simulink model "CIMA_LQ"  (R2023b)
settings: Solver=VariableStepAuto  StartTime=0.0  StopTime=30  RelTol=1e-6
values from neighbouring files (symbols this model uses):
  A = J_eq    [CIMA_Control_routine.m]
  a = 10    [CIMA_Classification_Stab_Equilibrium.m]    (also in CIMA_Control_routine.m)
  B = [1;0]    [CIMA_Control_routine.m]
  b = b_vec(i)    [CIMA_Classification_Stab_Equilibrium.m]    (also in CIMA_Control_routine.m = 2)
  C = eye(2)    [CIMA_Control_routine.m]
  D = zeros(2,1)    [CIMA_Control_routine.m]
  Eq = [x1_eq;x2_eq]    [CIMA_Control_routine.m]
  Ki = K(3)    [CIMA_Control_routine.m]
  Kp = K(1:2)    [CIMA_Control_routine.m]
  x0 = [x1_eq+0.5; x2_eq+0.2]    [CIMA_Control_routine.m]
settings Model: Creator=user  LastModifiedBy=user

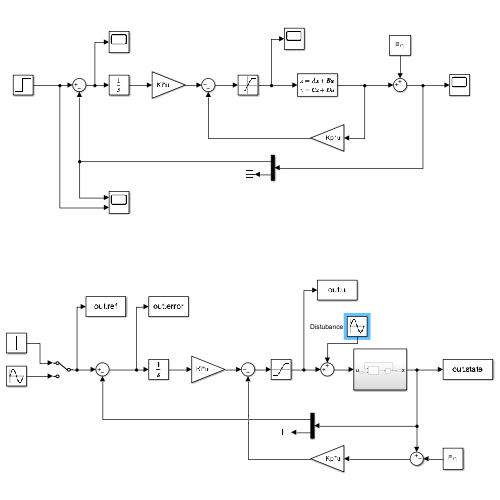
[thumbnail: Simulink's stored preview of the top-level diagram]
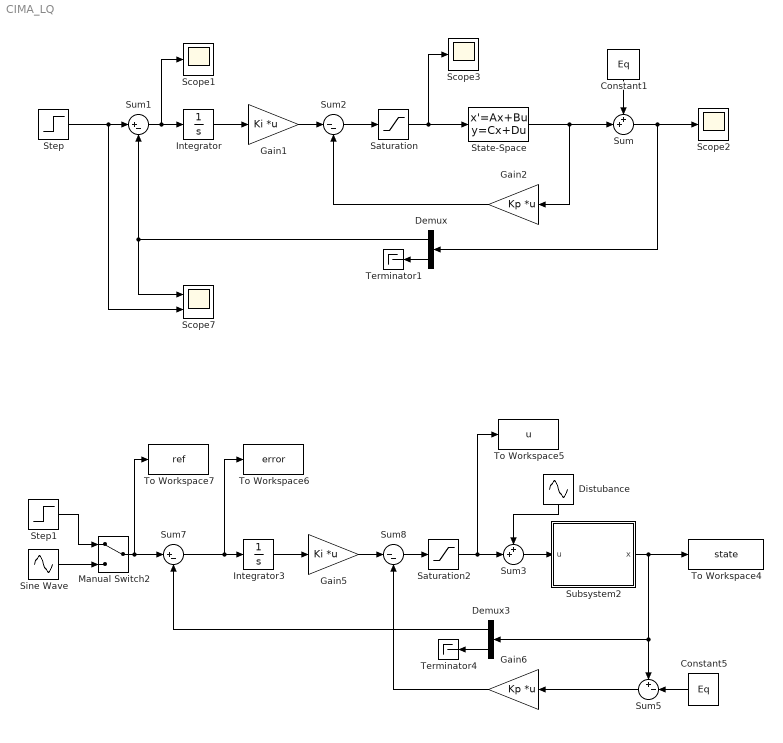
== system CIMA_LQ ==
  Constant1 : Constant  Value=Eq
  Constant5 : Constant  Value=Eq
  Demux : Demux  Outputs=2
  Demux3 : Demux  Outputs=2
  Distubance : Sin  Amplitude=0.3*0  SampleTime=0
  Gain1 : Gain  Gain=Ki  Multiplication=Matrix(K*u)
  Gain2 : Gain  Gain=Kp  Multiplication=Matrix(K*u)
  Gain5 : Gain  Gain=Ki  Multiplication=Matrix(K*u)
  Gain6 : Gain  Gain=Kp  Multiplication=Matrix(K*u)
  Integrator : Integrator
  Integrator3 : Integrator
  Manual Switch2 : ManualSwitch
  Saturation : Saturate  UpperLimit=20  LowerLimit=0
  Saturation2 : Saturate  UpperLimit=20  LowerLimit=0
  Scope1 : Scope
  Scope2 : Scope
  Scope3 : Scope
  Scope7 : Scope  NumInputPorts=2
  Sine Wave : Sin  Amplitude=0.5  Bias=5  Frequency=2  SampleTime=0
  State-Space : StateSpace  A=A  B=B  C=C  D=D  InitialCondition=x0-Eq  ParameterTunability=Optimized
  Step : Step  Time=0  After=5  SampleTime=0
  Step1 : Step  Time=0  After=5  SampleTime=0
  Subsystem2 : Subsystem
  Sum : Sum  Inputs=++|
  Sum1 : Sum  Inputs=|+-
  Sum2 : Sum  Inputs=|--
  Sum3 : Sum  Inputs=++|
  Sum5 : Sum  Inputs=+-|
  Sum7 : Sum  Inputs=|+-
  Sum8 : Sum  Inputs=|--
  Terminator1 : Terminator
  Terminator4 : Terminator
  To Workspace4 : ToWorkspace  VariableName=state  SaveFormat=Structure With Time  SampleTime=-1
  To Workspace5 : ToWorkspace  VariableName=u  SaveFormat=Structure With Time  SampleTime=-1
  To Workspace6 : ToWorkspace  VariableName=error  SaveFormat=Structure With Time  SampleTime=-1
  To Workspace7 : ToWorkspace  VariableName=ref  SaveFormat=Structure With Time  SampleTime=-1
  wires:
  Integrator/1 -> Gain1/1
  Sum2/1 -> Saturation/1
  Demux/1 -> Sum1/2, Scope7/1
  Gain1/1 -> Sum2/1
  Gain2/1 -> Sum2/2
  Sum/1 -> Scope2/1, Demux/1
  Sum1/1 -> Scope1/1, Integrator/1
  Demux/2 -> Terminator1/1
  Step/1 -> Scope7/2, Sum1/1
  Constant1/1 -> Sum/1
  State-Space/1 -> Gain2/1, Sum/2
  Saturation/1 -> State-Space/1, Scope3/1
  Demux3/1 -> Sum7/2
  Gain5/1 -> Sum8/1
  Gain6/1 -> Sum8/2
  Sum8/1 -> Saturation2/1
  Demux3/2 -> Terminator4/1
  Sum7/1 -> To Workspace6/1, Integrator3/1
  Manual Switch2/1 -> To Workspace7/1, Sum7/1
  Integrator3/1 -> Gain5/1
  Saturation2/1 -> To Workspace5/1, Sum3/2
  Step1/1 -> Manual Switch2/1
  Sine Wave/1 -> Manual Switch2/2
  Sum5/1 -> Gain6/1
  Constant5/1 -> Sum5/2
  Sum3/1 -> Subsystem2/1(u)
  Distubance/1 -> Sum3/1
  Subsystem2/1(x) -> To Workspace4/1, Demux3/1, Sum5/1

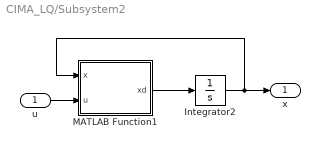
== system CIMA_LQ/Subsystem2 ==
  u : Inport
  Integrator2 : Integrator  InitialCondition=x0  UpperSaturationLimit=18
  MATLAB Function1 : MATLAB Function  TreatAsAtomicUnit=on
  x : Outport
  wires:
  MATLAB Function1/1(xd) -> Integrator2/1
  Integrator2/1 -> x/1, MATLAB Function1/1(x)
  u/1 -> MATLAB Function1/2(u)

== matlab function CIMA_LQ/Subsystem2/MATLAB Function1 ==
  data: x input; u input; xd output; a parameter; b parameter
function xd = cima(x, u, a, b)

xd1 = a -x(1) - 4*x(1)*x(2)/(1 + x(1)^2) + u; 
xd2 = b*x(1)*(1 - x(2)/(1 + x(1)^2)); 

% Parameter uncertanties 10%
%xd1 = 0.9*a -x(1) - 4*x(1)*x(2)/(1 + x(1)^2) + u; 
%xd2 = 1.1*b*x(1)*(1 - x(2)/(1 + x(1)^2)); 

% Parameter uncertanties 20%
%xd1 = 1.2*a -x(1) - 4*x(1)*x(2)/(1 + x(1)^2) + u; 
%xd2 = 0.8*b*x(1)*(1 - x(2)/(1 + x(1)^2));

xd = [xd1;xd2];
